simulink model "flo4_2018a"  (R2018a)
settings: Solver=ode45  StartTime=0.0  StopTime=inf  FixedStep=0.01  RelTol=1e-3  EnableMultiTasking=on
settings Model: EnablePacing=on  Creator=Florian  LastModifiedBy=Florian
settings SolverCC: AutoInsertRateTranBlk=on
settings DataIOCC: LimitDataPoints=on  ReturnWorkspaceOutputs=on
settings OptimizationCC: LifeSpan=inf
settings DebuggingCC: AllowSymbolicDim=off  SFUnexpectedBacktrackingDiag=warning  SFNoUnconditionalDefaultTransitionDiag=warning  SFExecutionAtInitializationDiag=none  SFMachineParentedDataDiag=error
settings CodeAppCC: StateflowObjectComments=on
settings GRTTargetCC: TargetLangStandard=C89/C90 (ANSI)
settings ConfigComp: CovMetricSettings=dw  CovSaveCumulativeToWorkspaceVar=on  CovSaveSingleToWorkspaceVar=on  CovExternalEMLEnable=off  CovSFcnEnable=off

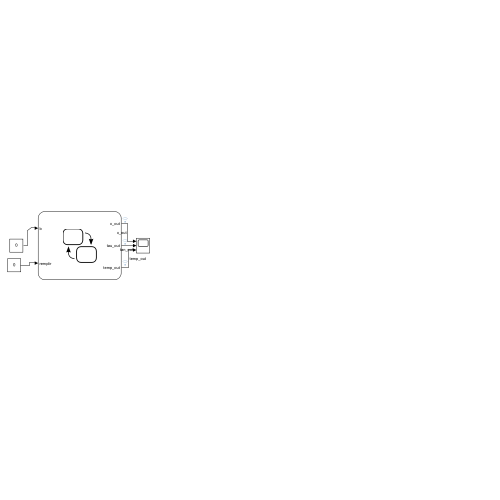
[thumbnail: Simulink's stored preview of the top-level diagram]
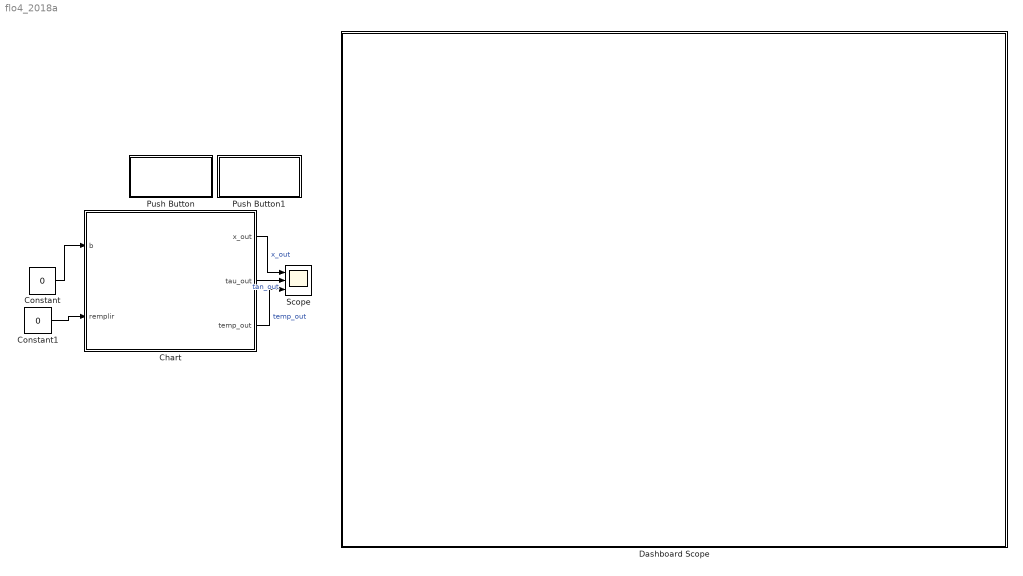
== system flo4_2018a ==
  Chart : Stateflow chart  TreatAsAtomicUnit=on
  Constant : Constant  Value=0
  Constant1 : Constant  Value=0
  Dashboard Scope : Subsystem  DialogController=hmiCreateDDGDialog  IsWebBlock=on  mask(MWDashboardBlock){webBlockId=7a4abf14-7aee-4baf-bde4-6e7067d9f8c5, webBlockType=sdiscope, ShowInLibBrowser=on, ShowInitialText=on, HMISrcModelName=flo4_2018a}
      mask prompts: webBlockId "WebBlock Id"; webBlockType "WebBlock Type"; HMISrcModelName "Source Model"
      mask help: Traces signals on the dashboard scope during simulation.
      mask Help: helpview([docroot '/mapfiles/simulink.map'], 'hmi_scope')
      mask Display:
      | if strcmp(get_param(bdroot(gcb),'BlockDiagramType'),'library')
      |  image([(matlabroot) '/toolbox/simulink/hmi/icons/SDIScope.png'])
      | end
  Push Button : Subsystem  DialogController=hmiCreateDDGDialog  IsWebBlock=on  mask(MWDashboardBlock){webBlockId=8f05e875-1d3c-4647-8ed1-9d7336bca1fd, webBlockType=pushbutton, ShowInLibBrowser=on, ShowInitialText=on, HMISrcModelName=flo4_2018a}
      mask prompts: webBlockId "WebBlock Id"; webBlockType "WebBlock Type"; HMISrcModelName "Source Model"
      mask help: Change the value of a variable or tunable parameter using a button. You can configure the button to respond to a click by momentarily changing the value until you release or by latching the value until you click again.
      mask Help: helpview([docroot '/mapfiles/simulink.map'], 'hmi_pushbutton')
      mask Display:
      | if strcmp(get_param(bdroot(gcb),'BlockDiagramType'),'library')
      |  image([(matlabroot) '/toolbox/simulink/hmi/icons/PushButton.png'])
      | end
  Push Button1 : Subsystem  DialogController=hmiCreateDDGDialog  IsWebBlock=on  mask(MWDashboardBlock){webBlockId=388728a7-19fe-43c9-83ef-abc074d747f2, webBlockType=pushbutton, ShowInLibBrowser=on, ShowInitialText=on, HMISrcModelName=flo4_2018a}
      mask prompts: webBlockId "WebBlock Id"; webBlockType "WebBlock Type"; HMISrcModelName "Source Model"
      mask help: Change the value of a variable or tunable parameter using a button. You can configure the button to respond to a click by momentarily changing the value until you release or by latching the value until you click again.
      mask Help: helpview([docroot '/mapfiles/simulink.map'], 'hmi_pushbutton')
      mask Display:
      | if strcmp(get_param(bdroot(gcb),'BlockDiagramType'),'library')
      |  image([(matlabroot) '/toolbox/simulink/hmi/icons/PushButton.png'])
      | end
  Scope : Scope  NumInputPorts=3
  wires:
  Chart/1(x_out) -> Scope/1  "x_out"
  Chart/2(tau_out) -> Scope/2  "tan_out"
  Constant/1 -> Chart/1(b)
  Constant1/1 -> Chart/2(remplir)
  Chart/3(temp_out) -> Scope/3  "temp_out"

== system flo4_2018a/Dashboard Scope ==

== system flo4_2018a/Push Button ==

== system flo4_2018a/Push Button1 ==

== stateflow chart flo4_2018a/Chart ==
  settings: updateMethod=CONTINUOUS  executeAtInitialization=1  initializeOutput=1
  state Q0
    du:
    %derivative
    x_dot=0;
    tau_dot=0;
    theta_dot = -(beta*(x_max-x) + k)*(theta-temp_amb);
    %output
    x_out = x;
    tau_out = tau;
    temp_out = theta;
  state Q1
    du:
    %derivative
    x_dot=-alpha;
    tau_dot=1;
    theta_dot = -(beta*(x_max-x) + k) * (theta-temp_amb);
    %output
    x_out = x;
    tau_out = tau;
    temp_out = theta;
  state Q02
    du:
    %derivative
    x_dot=0;
    tau_dot=0;
    theta_dot=gamma;
    %output
    x_out = x;
    tau_out = tau;
    temp_out = theta;
  state Q03
    du:
    %derivative
    x_dot=0;
    tau_dot=0;
    theta_dot=gamma;
    %output
    x_out = x;
    tau_out = tau;
    temp_out = theta;
  (default) -> Q0 : {x =100
      | tau = 0
      | theta = temp_amb}
  Q0 -> Q0 [order 3] : [x <= x_min && remplir]{x = x_max}
  Q0 -> Q1 [order 1] : [b && x > x_min && theta > 70]{tau = 0}
  Q1 -> Q0 : [tau >= tau_max || x <= 0]
  Q0 -> Q02 [order 2] : [theta <= 70 && x > x_min]
  Q02 -> Q0 [order 1] : [theta >= 80]
  Q03 -> Q1 : [theta >= 75]{tau = 0}
  Q02 -> Q03 [order 2] : [b && x > x_min && theta < 80]
  data: x local double; tau local double; x_out output double size=1; tau_out output double size=1; tau_max constant double =4; alpha constant double =3; b input; x_max local =100; remplir input; theta local; temp_out output; beta constant double =0.0001; k constant double =0.001; x_min local =12; temp_amb local =25; gamma constant double =1
  data x settings: updateMethod=SF_CONTINUOUS_TIME_DATA
  data tau settings: updateMethod=SF_CONTINUOUS_TIME_DATA
  data x_max settings: updateMethod=SF_CONTINUOUS_TIME_DATA
  data theta settings: updateMethod=SF_CONTINUOUS_TIME_DATA
  data x_min settings: updateMethod=SF_CONTINUOUS_TIME_DATA
